simulink model "failureInputReadHex"  (R2024a)
settings: configuration reference "standardSILConfiguraitonParams" (kept outside this file)
undefined symbols (not defined in the file): EnumHexFailureType
libraries: simulink x7
settings Model: Creator=jerem  LastModifiedBy=jerem
settings ConfigSetRef: SourceName=standardSILConfiguraitonParams  SourceLocation=Base Workspace

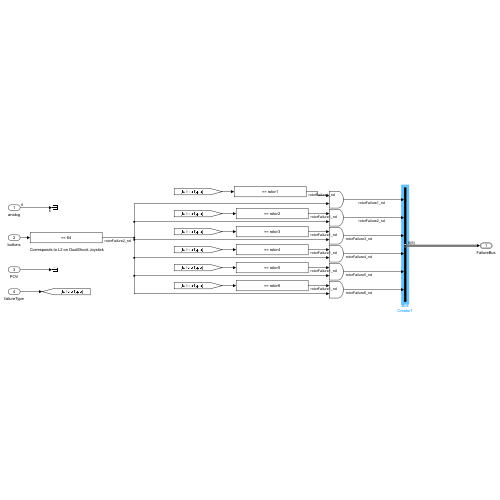
[thumbnail: Simulink's stored preview of the top-level diagram]
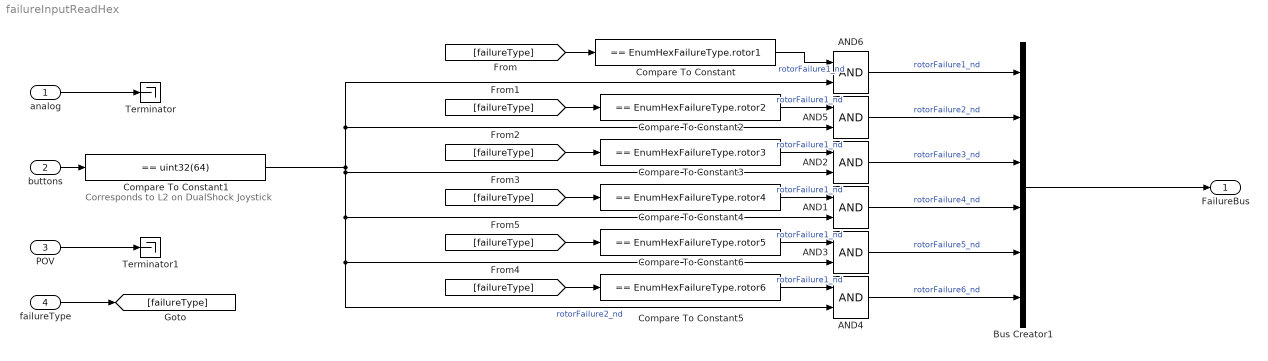
== system failureInputReadHex ==
  note: Corresponds to L2 on DualShock Joystick
  analog : Inport  PortDimensions=6
  buttons : Inport  Port=2  OutDataTypeStr=uint32
  POV : Inport  Port=3
  failureType : Inport  Port=4  OutDataTypeStr=Enum:EnumHexFailureType
  AND{1..6} (6 alike) : Logic  IconShape=distinctive  AllPortsSameDT=off  OutDataTypeStr=boolean
  Bus Creator1 : BusCreator  Inputs=6  OutDataTypeStr=Bus: FailureBus
  Compare To Constant : simulink/Logic and Bit Operations/Compare To Constant  relop===  const=EnumHexFailureType.rotor1  OutDataTypeStr=boolean
  Compare To Constant1 : simulink/Logic and Bit Operations/Compare To Constant  relop===  const=uint32(64)  OutDataTypeStr=boolean
  Compare To Constant2 : simulink/Logic and Bit Operations/Compare To Constant  relop===  const=EnumHexFailureType.rotor2  OutDataTypeStr=boolean
  Compare To Constant3 : simulink/Logic and Bit Operations/Compare To Constant  relop===  const=EnumHexFailureType.rotor3  OutDataTypeStr=boolean
  Compare To Constant4 : simulink/Logic and Bit Operations/Compare To Constant  relop===  const=EnumHexFailureType.rotor4  OutDataTypeStr=boolean
  Compare To Constant5 : simulink/Logic and Bit Operations/Compare To Constant  relop===  const=EnumHexFailureType.rotor6  OutDataTypeStr=boolean
  Compare To Constant6 : simulink/Logic and Bit Operations/Compare To Constant  relop===  const=EnumHexFailureType.rotor5  OutDataTypeStr=boolean
  Terminator : Terminator
  Terminator1 : Terminator
  FailureBus : Outport  OutDataTypeStr=Bus: FailureBus
  wires:
  analog/1 -> Terminator/1
  POV/1 -> Terminator1/1
  Bus Creator1/1 -> FailureBus/1
  AND5/1 -> Bus Creator1/2  "rotorFailure2_nd"
  AND2/1 -> Bus Creator1/3  "rotorFailure3_nd"
  AND1/1 -> Bus Creator1/4  "rotorFailure4_nd"
  AND3/1 -> Bus Creator1/5  "rotorFailure5_nd"
  AND4/1 -> Bus Creator1/6  "rotorFailure6_nd"
  failureType/1 -> [failureType]
  buttons/1 -> Compare To Constant1/1
  [failureType] -> Compare To Constant/1
  AND6/1 -> Bus Creator1/1  "rotorFailure1_nd"
  [failureType] -> Compare To Constant2/1
  Compare To Constant2/1 -> AND5/1  "rotorFailure1_nd"
  Compare To Constant/1 -> AND6/1  "rotorFailure1_nd"
  Compare To Constant1/1 -> AND5/2, AND6/2, AND1/2, AND3/2, AND4/2, AND2/2  "rotorFailure2_nd"
  [failureType] -> Compare To Constant3/1
  Compare To Constant3/1 -> AND2/1  "rotorFailure1_nd"
  [failureType] -> Compare To Constant4/1
  Compare To Constant4/1 -> AND1/1  "rotorFailure1_nd"
  [failureType] -> Compare To Constant5/1
  Compare To Constant5/1 -> AND4/1  "rotorFailure1_nd"
  [failureType] -> Compare To Constant6/1
  Compare To Constant6/1 -> AND3/1  "rotorFailure1_nd"
